simulink model "lab1"  (R2022a)
settings: Solver=VariableStepAuto  StartTime=0.0  StopTime=10.0  RelTol=1e-3
settings Model: Creator=Dubov  LastModifiedBy=Dubov

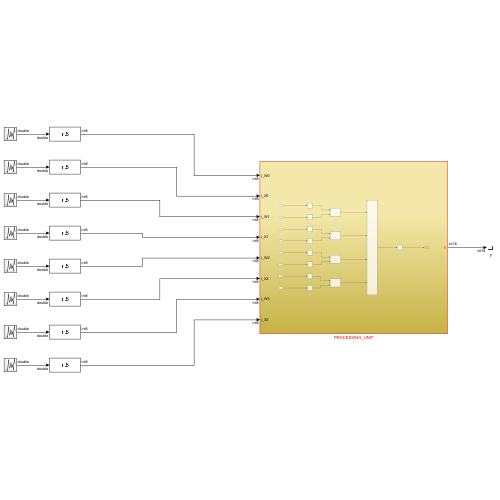
[thumbnail: Simulink's stored preview of the top-level diagram]
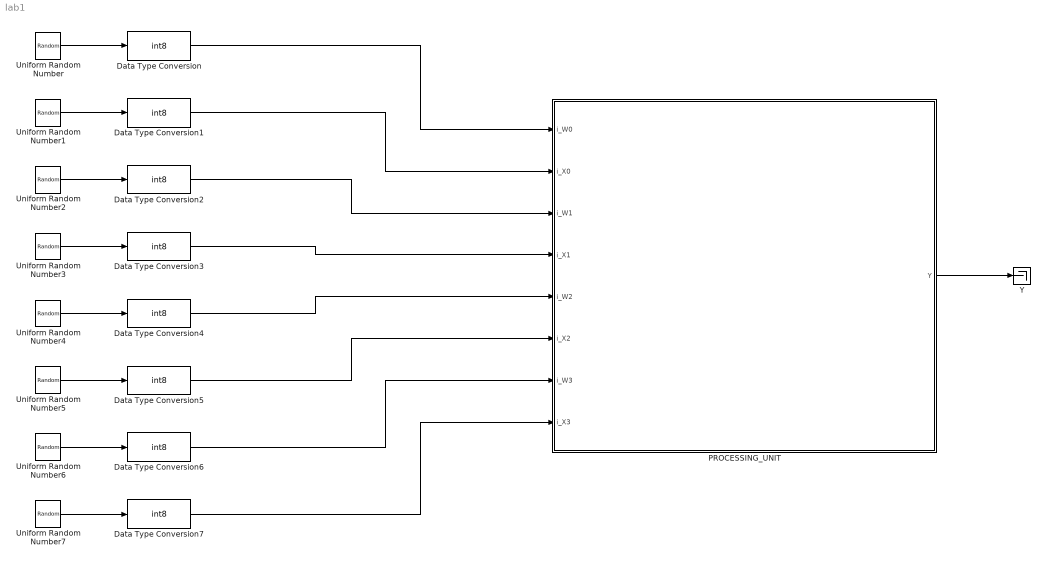
== system lab1 ==
  Data Type Conversion{,1..7} (8 alike) : DataTypeConversion  OutDataTypeStr=int8  SaturateOnIntegerOverflow=off  RndMeth=Floor
  PROCESSING_UNIT : Subsystem
  Uniform Random Number : UniformRandomNumber  Minimum=0  Maximum=2^8-1  Seed=5  SampleTime=1
  Uniform Random Number1 : UniformRandomNumber  Minimum=0  Maximum=2^8-1  Seed=6  SampleTime=1
  Uniform Random Number2 : UniformRandomNumber  Minimum=0  Maximum=2^8-1  Seed=7  SampleTime=1
  Uniform Random Number3 : UniformRandomNumber  Minimum=0  Maximum=2^8-1  Seed=8  SampleTime=1
  Uniform Random Number4 : UniformRandomNumber  Minimum=0  Maximum=2^8-1  Seed=9  SampleTime=1
  Uniform Random Number5 : UniformRandomNumber  Minimum=0  Maximum=2^8-1  Seed=10  SampleTime=1
  Uniform Random Number6 : UniformRandomNumber  Minimum=0  Maximum=2^8-1  Seed=11  SampleTime=1
  Uniform Random Number7 : UniformRandomNumber  Minimum=0  Maximum=2^8-1  Seed=12  SampleTime=1
  Y : Terminator
  wires:
  Uniform Random Number/1 -> Data Type Conversion/1
  Uniform Random Number1/1 -> Data Type Conversion1/1
  Uniform Random Number2/1 -> Data Type Conversion2/1
  Uniform Random Number3/1 -> Data Type Conversion3/1
  Uniform Random Number4/1 -> Data Type Conversion4/1
  Uniform Random Number5/1 -> Data Type Conversion5/1
  Uniform Random Number6/1 -> Data Type Conversion6/1
  Uniform Random Number7/1 -> Data Type Conversion7/1
  Data Type Conversion/1 -> PROCESSING_UNIT/1(i_W0)
  Data Type Conversion1/1 -> PROCESSING_UNIT/2(i_X0)
  Data Type Conversion2/1 -> PROCESSING_UNIT/3(i_W1)
  Data Type Conversion3/1 -> PROCESSING_UNIT/4(i_X1)
  Data Type Conversion4/1 -> PROCESSING_UNIT/5(i_W2)
  Data Type Conversion5/1 -> PROCESSING_UNIT/6(i_X2)
  Data Type Conversion6/1 -> PROCESSING_UNIT/7(i_W3)
  Data Type Conversion7/1 -> PROCESSING_UNIT/8(i_X3)
  PROCESSING_UNIT/1(Y) -> Y/1

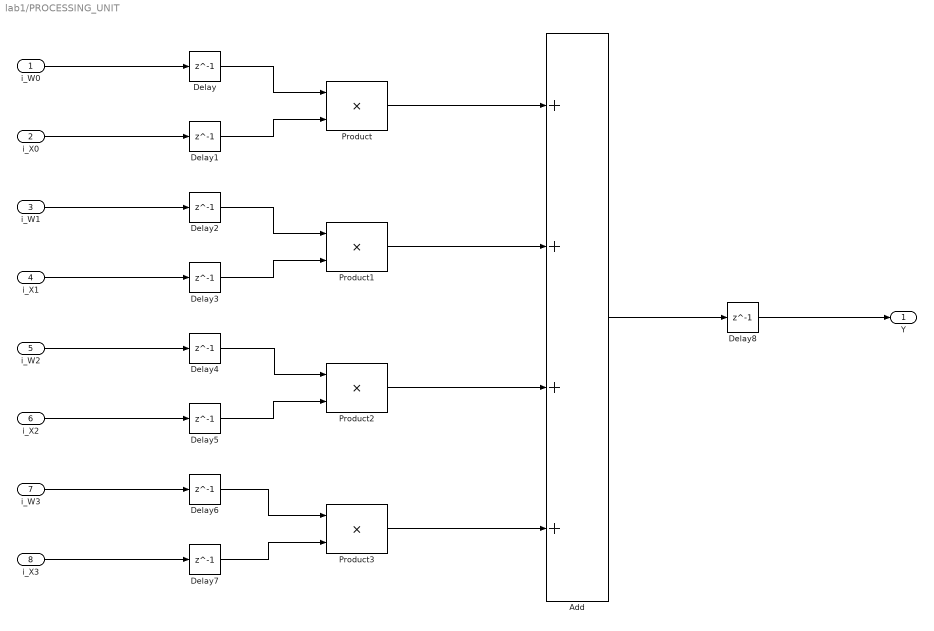
== system lab1/PROCESSING_UNIT ==
  i_W0 : Inport  OutDataTypeStr=int8
  i_X0 : Inport  Port=2  OutDataTypeStr=int8
  i_W1 : Inport  Port=3  OutDataTypeStr=int8
  i_X1 : Inport  Port=4  OutDataTypeStr=int8
  i_W2 : Inport  Port=5  OutDataTypeStr=int8
  i_X2 : Inport  Port=6  OutDataTypeStr=int8
  i_W3 : Inport  Port=7  OutDataTypeStr=int8
  i_X3 : Inport  Port=8  OutDataTypeStr=int8
  Add : Sum  Inputs=++++  AccumDataTypeStr=int16
  Delay{,1..8} (9 alike) : Delay  DelayLength=1  InitialCondition=0
  Product{,1..3} (4 alike) : Product  OutDataTypeStr=int16
  Y : Outport  OutDataTypeStr=int16
  wires:
  Add/1 -> Delay8/1
  i_X3/1 -> Delay7/1
  Delay7/1 -> Product3/2
  Product2/1 -> Add/3
  Delay4/1 -> Product2/1
  Product3/1 -> Add/4
  Delay3/1 -> Product1/2
  Delay/1 -> Product/1
  Delay2/1 -> Product1/1
  Delay6/1 -> Product3/1
  Delay1/1 -> Product/2
  Product/1 -> Add/1
  Delay5/1 -> Product2/2
  Product1/1 -> Add/2
  i_W1/1 -> Delay2/1
  i_W0/1 -> Delay/1
  Delay8/1 -> Y/1
  i_X0/1 -> Delay1/1
  i_X2/1 -> Delay5/1
  i_X1/1 -> Delay3/1
  i_W2/1 -> Delay4/1
  i_W3/1 -> Delay6/1
